simulink model "kinSwCtrl"  (R2015a)
settings: Solver=ode45  StartTime=0.0  StopTime=sim_t  RelTol=1e-3
InitFcn:
  | set_kinSwCtrl;
values from neighbouring files (symbols this model uses):
  COM_x_dx = -[0.05 -1]    [set_kinSwCtrl.m]
  COM_y_dy = -[0.05 0]    [set_kinSwCtrl.m]
  kinSw_footx_tgt = kinSw_len_tgt*cos(kinSw_alpha_tgt)    [set_kinSwCtrl.m]
  kinSw_footy_tgt = -0.05    [set_kinSwCtrl.m]
  kinSw_min_f_duration = kinSw_time_del*0.85    (= 0.425)    [set_kinSwCtrl.m]    (also in set_kinSwCtrl2.m)
  kinSw_parabolic_z_retraction = 0.9-kinSw_len_tgt    (= 0.1)    [set_kinSwCtrl.m]
  kinSw_time_del = 0.5    [set_kinSwCtrl.m]    (also in set_kinSwCtrl2.m)
  kinSw_z_land = kinSw_len_tgt*sin(kinSw_alpha_tgt)    [set_kinSwCtrl.m]
  test_t_SwStart = 0.001    [set_kinSwCtrl.m]    (also in set_kinSwCtrl2.m)
  z_dz_foot2com = [0.8 0]    [set_kinSwCtrl.m]
libraries: simulink x2
settings Model: Creator=smsong  LastModifiedBy=smsong

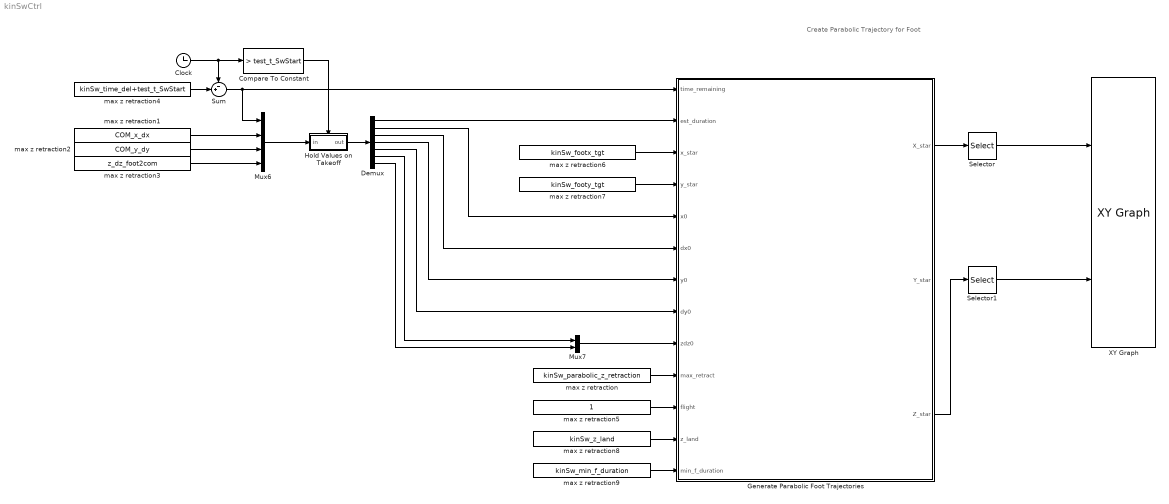
== system kinSwCtrl ==
  note: Create Parabolic
      | Trajectory for Foot
  Clock : Clock
  Compare To Constant : simulink/Logic and Bit Operations/Compare To Constant  relop=>  const=test_t_SwStart  OutDataTypeStr=boolean  ZeroCross=off
  Demux : Demux  Outputs=7
  Generate Parabolic Foot Trajectories : MATLAB Function  TreatAsAtomicUnit=on
  Hold Values on Takeoff : Subsystem
  Mux6 : Mux
  Mux7 : Mux  Inputs=2
  Selector : Selector  InputPortWidth=3
  Selector1 : Selector  InputPortWidth=3
  Sum : Sum  Inputs=-+|
  XY Graph : simulink/Sinks/XY Graph  xmin=-1  xmax=1  ymin=-1  ymax=1  st=-1
  max z retraction : Constant  Value=kinSw_parabolic_z_retraction
  max z retraction1 : Constant  Value=COM_x_dx
  max z retraction2 : Constant  Value=COM_y_dy
  max z retraction3 : Constant  Value=z_dz_foot2com
  max z retraction4 : Constant  Value=kinSw_time_del+test_t_SwStart
  max z retraction5 : Constant
  max z retraction6 : Constant  Value=kinSw_footx_tgt
  max z retraction7 : Constant  Value=kinSw_footy_tgt
  max z retraction8 : Constant  Value=kinSw_z_land
  max z retraction9 : Constant  Value=kinSw_min_f_duration
  wires:
  Demux/1 -> Generate Parabolic Foot Trajectories/2(est_duration)
  Mux7/1 -> Generate Parabolic Foot Trajectories/9(zdz0)
  max z retraction/1 -> Generate Parabolic Foot Trajectories/10(max_retract)
  Mux6/1 -> Hold Values on Takeoff/1(in)
  Hold Values on Takeoff/1(out) -> Demux/1
  max z retraction1/1 -> Mux6/2
  Generate Parabolic Foot Trajectories/1(X_star) -> Selector/1
  max z retraction6/1 -> Generate Parabolic Foot Trajectories/3(x_star)
  max z retraction2/1 -> Mux6/3
  Sum/1 -> Mux6/1, Generate Parabolic Foot Trajectories/1(time_remaining)
  max z retraction7/1 -> Generate Parabolic Foot Trajectories/4(y_star)
  max z retraction5/1 -> Generate Parabolic Foot Trajectories/11(flight)
  Demux/2 -> Generate Parabolic Foot Trajectories/5(x0)
  Demux/3 -> Generate Parabolic Foot Trajectories/6(dx0)
  Demux/4 -> Generate Parabolic Foot Trajectories/7(y0)
  Demux/5 -> Generate Parabolic Foot Trajectories/8(dy0)
  Demux/6 -> Mux7/1
  Demux/7 -> Mux7/2
  max z retraction3/1 -> Mux6/4
  max z retraction4/1 -> Sum/2
  Clock/1 -> Compare To Constant/1, Sum/1
  Compare To Constant/1 -> Hold Values on Takeoff/Trigger
  max z retraction8/1 -> Generate Parabolic Foot Trajectories/12(z_land)
  max z retraction9/1 -> Generate Parabolic Foot Trajectories/13(min_f_duration)
  Selector/1 -> XY Graph/1
  Selector1/1 -> XY Graph/2
  Generate Parabolic Foot Trajectories/3(Z_star) -> Selector1/1

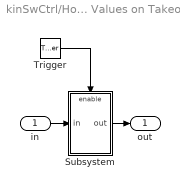
== system kinSwCtrl/Hold Values on Takeoff ==
  in : Inport
  Trigger : TriggerPort  ShowOutputPort=on  PortDimensions=1
  Subsystem : Subsystem
  out : Outport
  wires:
  Trigger/1 -> Subsystem/Enable
  Subsystem/1(out) -> out/1
  in/1 -> Subsystem/1(in)

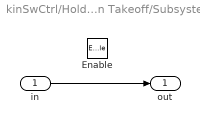
== system kinSwCtrl/Hold Values on Takeoff/Subsystem ==
  in : Inport
  Enable : EnablePort
  out : Outport
  wires:
  in/1 -> out/1

== matlab function kinSwCtrl/Generate Parabolic Foot Trajectories ==
  data: time_remaining input; est_duration input; x_star input; y_star input; x0 input; dx0 input; y0 input; dy0 input; zdz0 input; max_retract input; flight input; X_star output size=3; Y_star output size=3; Z_star output size=3; z_land input; min_f_duration input
%% Parabolic trajectory generation for x, y, and z
% est_duration: estimated flight time
% time_remaining: time until estimated touchdown
% stance: 1 if in stance, 0 otherwise
% x_star: desired x for foot to COM
% y_star: desired y for foot to COM
% x0: x position at takeoff
% y0: y position at takeoff
% zdz0: [z, dz] at takeoff
% max_retract: how high to lift z for ground clearance
% z_land: nominal z height for landing
% min_f_duration: minimum trajectory time

function [X_star, Y_star, Z_star]  =  ...
          GenerateParabolicFootTrajectory(time_remaining, est_duration,  ...
                               x_star, y_star, x0, dx0, y0, dy0, zdz0, ...
                               max_retract,  flight, z_land, min_f_duration)

if ~flight
    X_star = [0;0;0];
    Y_star = [0;0;0];
    Z_star = [0;0;0];
    return;
end
                           
% we are solving for yawed coordinates xyz of com-foot in flight and
% converting them to joint angles

% estimate z ballistically
% z = z_dz_liftoff(1) + z_dz_liftoff(2)*t_flight -g/2*t_flight^2;
% dz = z_dz_liftoff(2) - g*t_flight;
% 
% z = com_xdx_ydy_zdz(5); dz = com_xdx_ydy_zdz(6);
% time_remaining = (-dz-sqrt(max(dz^2 - 4*g/2*(z_land-z), 0) ) )/ (-g); % ballistic estimate of landing


  % plan a traj from init to desired in estimated duration. Use a
  % discontinuous initial condition if estimated duration too short.
  duration = max(est_duration, min_f_duration);
  t_r = max(min(time_remaining, duration),0);
  % sweep a parabola from x0 to x_star with dx_end = -dx0
  dx_star = dx0;
  x_star_t = x_star + dx_star*t_r + (x0-x_star-dx_star*duration)*(t_r/duration)^2;
  dx_star_t = -dx_star - 2*(x0-x_star-dx_star*duration)*(t_r/duration^2);
  ddx_star_t =  2*(x0-x_star-dx_star*duration)*(1/duration^2);
  
  % same for y
  dy_star = dy0;
  y_star_t = y_star + dy_star*t_r + (y0-y_star-dy_star*duration)*(t_r/duration)^2;
  dy_star_t = -dy_star - 2*(y0-y_star-dy_star*duration)*(t_r/duration^2);
  ddy_star_t =  2*(y0-y_star-dy_star*duration)*(1/duration^2);
  
  % Zero out velocities when out of time
  if time_remaining < 0
    dx_star_t = 0; ddx_star_t = 0;
    dy_star_t = 0; ddy_star_t = 0;
  end 
  
  % split duration into thirds.  First segment: parabola from z0 to
  % max_retract.  Second and third segments, cos to landing.
  z0 = zdz0(1);
  dt3 = duration / 3;
  z_min = z_land - max_retract;
  if t_r > 2*dt3;
    z_star_t = z_min + (z0-z_min)*((t_r-2*dt3)/dt3)^2;
    dz_star_t = -(z0-z_min)*2*(t_r-2*dt3)/dt3/dt3;
    ddz_star_t = (z0-z_min)*2/dt3^2;
  else
    z_star_t = z_land + (z_min-z_land)/2*(1-cos(t_r/(2*dt3)*pi));
    dz_star_t = -(z_min-z_land)/2*sin(t_r/(2*dt3)*pi)*pi/(2*dt3);
    ddz_star_t = (z_min-z_land)/2*cos(t_r/(2*dt3)*pi)*(pi/(2*dt3))^2;
  end
  
  % track a sinusoidal z of amplitude max_retract, finishing a half-cycle by t_end
  X_star = [x_star_t; dx_star_t; ddx_star_t];
  Y_star = [y_star_t; dy_star_t; ddy_star_t];
  Z_star = [z_star_t; dz_star_t; ddz_star_t];
